simulink model "magnetometer_v010422"  (R2022a)
settings: Solver=VariableStepAuto  StartTime=0.0  StopTime=10.0  RelTol=1e-3
settings Model: Creator=kathe  LastModifiedBy=kathe
settings DataIOCC: ExternalInput=[m]  LoadExternalInput=on

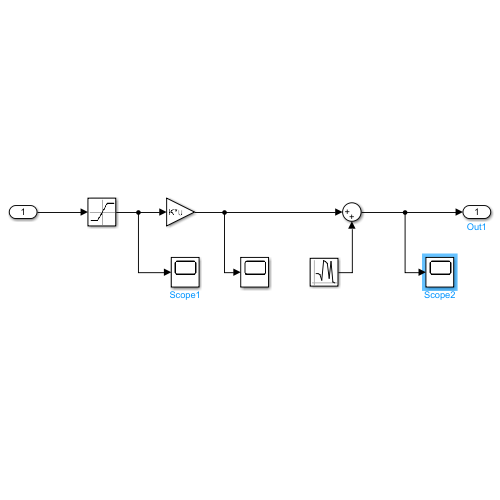
[thumbnail: Simulink's stored preview of the top-level diagram]
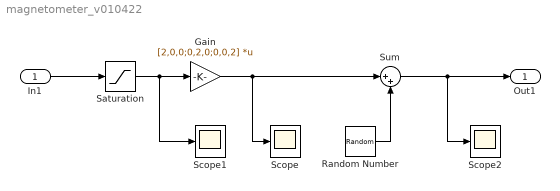
== system magnetometer_v010422 ==
  In1 : Inport  OutDataTypeStr=int8  PortDimensions=3
  Gain : Gain  Gain=[2,0,0;0,2,0;0,0,2]  Multiplication=Matrix(K*u)
  Random Number : RandomNumber  SampleTime=0.1
  Saturation : Saturate  UpperLimit=[70, 70, 70]  LowerLimit=[-70, -70, -70]
  Scope : Scope
  Scope1 : Scope
  Scope2 : Scope
  Sum : Sum  Inputs=|++
  Out1 : Outport
  wires:
  Gain/1 -> Sum/1, Scope/1
  In1/1 -> Saturation/1
  Saturation/1 -> Scope1/1, Gain/1
  Random Number/1 -> Sum/2
  Sum/1 -> Scope2/1, Out1/1
